simulink model "qss_saab93_test2"  (Simulink 6.4)
settings: Solver=VariableStepDiscrete  StartTime=0.0  StopTime=0  RelTol=1e-3
libraries: qss_tb_library x5
settings Model: LastModifiedBy=jofr
settings OptimizationCC: InlineInvariantSignals=on
settings DebuggingCC: StrictBusMsg=None

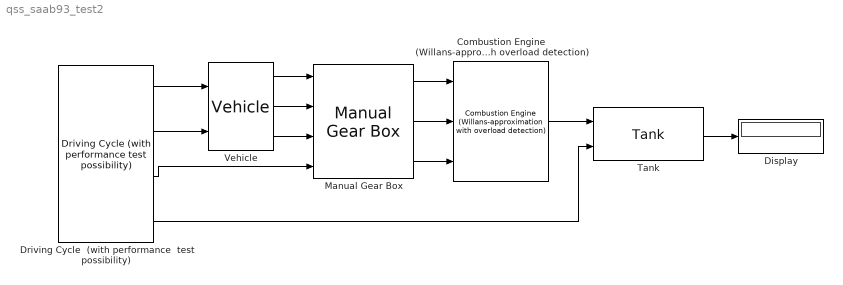
== system qss_saab93_test2 ==
  Combustion Engine (Willans-approximation  with overload detection) : qss_tb_library/Energy Converter/Combustion Engine (Willans-approximation  with overload detection)  Tag=combustion engine  SystemSampleTime=-1  engine_type=Otto  V_d=1.985  theta_CE=0.05  S=78  B=90  maxTorque=[177 4300]  maxPower=[96 6100]  w_CE_upper=700  w_CE_idle=105  P_CE_idle=2600  P_aux=300  e=0.46  PI=2  p_me0g=1  ENABLE_FUEL_CUTOFF=on  T_CE_cutoff=5  P_CE_cutoff=0
  Display : Display
  Driving Cycle  (with performance  test possibility) : qss_tb_library/Driving Cycle/Driving Cycle  (with performance  test possibility)  Tag=cycle  SystemSampleTime=-1  cyclenr=Europe: NEDC  stepsize=1  autostop=on  test=on  v_init=start_vel  v_end=end_vel  acc_constant=const_acc  gearon=upshift  gearoff=downshift
  Manual Gear Box : qss_tb_library/Gear System/Manual Gear Box  Tag=transmission  SystemSampleTime=-1  i_1=3.38  i_2=1.76  i_3=1.12  i_4=0.89  i_5=0.7  i_diff=4.45  e_GT=0.98  P_GT0=300  w_wheel_min=1
  Tank : qss_tb_library/Energy Source/Tank  Tag=tank  SystemSampleTime=-1  fuel=Gasoline  flag_cold_start=on
  Vehicle : qss_tb_library/Vehicle/Vehicle  Tag=vehicle  SystemSampleTime=-1  m_f=1295+80+100  mt2m_f=5  A_f=2  d_wheel=0.62  cw=0.3  mu=0.013
  wires:
  Driving Cycle  (with performance  test possibility)/1 -> Vehicle/1
  Vehicle/1 -> Manual Gear Box/1
  Vehicle/2 -> Manual Gear Box/2
  Driving Cycle  (with performance  test possibility)/2 -> Vehicle/2
  Manual Gear Box/1 -> Combustion Engine (Willans-approximation  with overload detection)/1
  Manual Gear Box/2 -> Combustion Engine (Willans-approximation  with overload detection)/2
  Manual Gear Box/3 -> Combustion Engine (Willans-approximation  with overload detection)/3
  Combustion Engine (Willans-approximation  with overload detection)/1 -> Tank/1
  Driving Cycle  (with performance  test possibility)/3 -> Manual Gear Box/4
  Driving Cycle  (with performance  test possibility)/4 -> Tank/2
  Tank/1 -> Display/1
  Vehicle/3 -> Manual Gear Box/3
